simulink model "inverse_pendulum"  (R2016a)
settings: Solver=FixedStepAuto  StartTime=0.0  StopTime=inf  FixedStep=1e-4  RelTol=1e-3
undefined symbols (not defined in the file or in its folder): sigbuilder_block
libraries: fuzblock x6, simulink x2
settings Model: Creator=Salar Basiri  LastModifiedBy=Salar Basiri

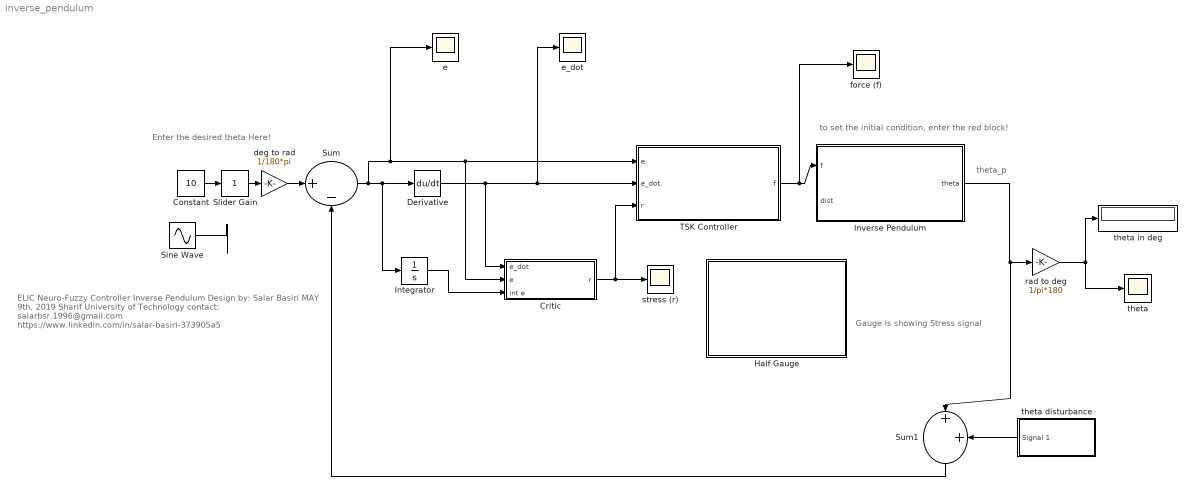
== system inverse_pendulum ==
  note: ELIC Neuro-Fuzzy Controller
      | Inverse Pendulum
      | Design by: Salar Basiri
      | MAY 9th, 2019
      | Sharif University of Technology
      | contact:
      | salarbsr.1996@gmail.com
      | https://www.linkedin.com/in/salar-basiri-373905a5
  note: to set the initial condition, enter the red block!
  note: Gauge is showing Stress signal
  note: Enter the desired theta Here!
  note: theta_p
  Constant : Constant  Value=10
  Critic : Subsystem
  Derivative : Derivative
  Half Gauge : Subsystem  DialogController=hmiCreateDDGDialog  IsWebBlock=on  mask(MWDashboardBlock){webBlockId=e21a16ba-fe41-4bad-9400-f35b9216ae1c, webBlockType=semicirculargauge, ShowInLibBrowser=on, ShowInitialText=on, HMISrcModelName=inverse_pendulum}
      mask prompts: webBlockId "WebBlock Id"; webBlockType "WebBlock Type"; HMISrcModelName "Source Model"
      mask Help: helpview([docroot '/mapfiles/simulink.map'], 'hmi_half_gauge')
      mask Display:
      | if strcmp(get_param(bdroot(gcb),'BlockDiagramType'), 'library')
      |     image([(matlabroot) '/toolbox/simulink/hmi/icons/SemicircularGauge.png']);
      | end
  Integrator : Integrator
  Inverse Pendulum : Subsystem
  Sine Wave : Sin  Amplitude=10  Frequency=5  SampleTime=0
  Slider Gain : simulink/Math Operations/Slider Gain  low=-1  gain=1  high=1
  Sum : Sum  Inputs=|+-
  Sum1 : Sum  Inputs=|++
  TSK Controller : Subsystem
  deg to rad : Gain  Gain=1/180*pi
  e : Scope
  e_dot : Scope
  force (f) : Scope
  rad to deg : Gain  Gain=1/pi*180
  stress (r) : Scope
  theta : Scope
  theta disturbance : Subsystem  Tag=STV Subsys  LoadFcn=sigbuilder_block('load');  StartFcn=sigbuilder_block('start');  StopFcn=sigbuilder_block('stop');  ClipboardFcn=sigbuilder_block('clipboard');  mask(Sigbuilder block){}
      mask help: Simulink:masks:SigbuilderBlock_MD
      mask init:
      | if ~strcmp(get_param(bdroot(gcbh),'SimulationStatus'),'stopped') tuvar = sigbuilder_block('maskInit'); end
      settings: CopyFcn=sigbuilder_block('copy');  DeleteFcn=sigbuilder_block('delete');  ModelCloseFcn=sigbuilder_block('modelClose');  PreSaveFcn=sigbuilder_block('preSave');  PauseFcn=sigbuilder_block('pause');  ContinueFcn=sigbuilder_block('continue');  NameChangeFcn=sigbuilder_block('namechange');  OpenFcn=sigbuilder_block('open',[6 30 1012.5 447.75 ]);  CloseFcn=sigbuilder_block('close');
      mask Display: plot(0, 0, 100, 100,[2, 2, 32, 32, 2], [68, 8, 8, 68, 68],[32, 2], [38, 38], [32, 19, 2],[53, 60, 44], [32, 17, 17, 2],[16, 16, 31, 31]);txt = getActiveGroup(gcbh);text(2, 100, txt,'verticalAlignment', 'top');
  theta in deg : Display
  wires:
  Inverse Pendulum/1(theta) -> Sum1/1, rad to deg/1
  Sum/1 -> Integrator/1, Derivative/1, e/1, Critic/2(e), TSK Controller/1(e)
  Derivative/1 -> Critic/1(e_dot), e_dot/1, TSK Controller/2(e_dot)
  TSK Controller/1(f) -> force (f)/1, Inverse Pendulum/1(f)
  rad to deg/1 -> theta/1, theta in deg/1
  deg to rad/1 -> Sum/1
  theta disturbance/1(Signal 1) -> Sum1/2
  Sum1/1 -> Sum/2
  Critic/1(r) -> TSK Controller/3(r), stress (r)/1
  Integrator/1 -> Critic/3(int e)
  Sine Wave/1 -> ?
  Slider Gain/1 -> deg to rad/1
  Constant/1 -> Slider Gain/1

== system inverse_pendulum/Critic ==
  e_dot : Inport
  e : Inport  Port=2
  int e : Inport  Port=3
  Constant : Constant  Value=20
  Constant1 : Constant  Value=5
  Constant2 : Constant  Value=10
  Product : Product
  Product1 : Product
  Product2 : Product
  Sum : Sum  Inputs=|+++
  r : Outport
  wires:
  Constant/1 -> Product/1
  e/1 -> Product/2
  e_dot/1 -> Product1/1
  Constant1/1 -> Product1/2
  Product/1 -> Sum/1
  Product1/1 -> Sum/2
  Sum/1 -> r/1
  int e/1 -> Product2/2
  Constant2/1 -> Product2/1
  Product2/1 -> Sum/3

== system inverse_pendulum/Half Gauge ==

== system inverse_pendulum/Inverse Pendulum ==
  note: set the initial conditions HERE!
  f : Inport
  dist : Inport  Port=2
  "Integrator, Second-Order" : SecondOrderIntegrator  ICX=0  ICDXDT=10/180*pi
  MATLAB Function : MATLAB Function  TreatAsAtomicUnit=on
  theta : Outport
  wires:
  "Integrator, Second-Order"/1 -> MATLAB Function/1(theta), theta/1
  "Integrator, Second-Order"/2 -> MATLAB Function/2(theta_p)
  f/1 -> MATLAB Function/3(f)
  MATLAB Function/1(theta_pp) -> "Integrator, Second-Order"/1
  dist/1 -> MATLAB Function/4(dist)

== system inverse_pendulum/TSK Controller ==
  e : Inport
  e_dot : Inport  Port=2
  r : Inport  Port=3
  Bus Creator : BusCreator  Inputs=3
  Subsystem : Subsystem
  Subsystem1 : Subsystem
  Subsystem10 : Subsystem
  Subsystem2 : Subsystem
  Subsystem3 : Subsystem
  Subsystem4 : Subsystem
  Subsystem5 : Subsystem
  Subsystem6 : Subsystem
  Subsystem7 : Subsystem
  Subsystem8 : Subsystem
  Subsystem9 : Subsystem
  Sum : Sum  Inputs=|+++++++++
  force limit : Saturate  UpperLimit=5  LowerLimit=-5
  f : Outport
  wires:
  e/1 -> Subsystem2/3(e), Subsystem8/3(e), Subsystem9/3(e), Subsystem10/3(e), Subsystem7/3(e), Subsystem6/3(e), Subsystem5/3(e), Subsystem4/3(e), Subsystem3/3(e), Subsystem1/2(e), Subsystem/1(e)
  e_dot/1 -> Subsystem3/4(e_dot), Subsystem5/4(e_dot), Subsystem6/4(e_dot), Subsystem7/4(e_dot), Subsystem8/4(e_dot), Subsystem10/4(e_dot), Subsystem9/4(e_dot), Subsystem4/4(e_dot), Subsystem2/4(e_dot), Subsystem/2(e_dot), Subsystem1/3(e_dot)
  r/1 -> Subsystem1/1(r)
  Subsystem/1(rule1) -> Subsystem2/1(myu)
  Subsystem1/1(a) -> Bus Creator/1
  Subsystem1/2(b) -> Bus Creator/2
  Subsystem1/3(c) -> Bus Creator/3
  Bus Creator/1 -> Subsystem5/2("mux "), Subsystem6/2("mux "), Subsystem8/2("mux "), Subsystem10/2("mux "), Subsystem9/2("mux "), Subsystem7/2("mux "), Subsystem3/2("mux "), Subsystem4/2("mux "), Subsystem2/2("mux ")
  Subsystem/2(rule2) -> Subsystem3/1(myu)
  Subsystem/3(rule3) -> Subsystem4/1(myu)
  Subsystem/4(rule4) -> Subsystem5/1(myu)
  Subsystem/5(rule5) -> Subsystem6/1(myu)
  Subsystem/6(rule6) -> Subsystem7/1(myu)
  Subsystem/7(rule7) -> Subsystem8/1(myu)
  Subsystem/8(rule8) -> Subsystem9/1(myu)
  Subsystem/9(rule9) -> Subsystem10/1(myu)
  Subsystem3/1(f) -> Sum/1
  Subsystem4/1(f) -> Sum/2
  Subsystem5/1(f) -> Sum/3
  Subsystem6/1(f) -> Sum/4
  Subsystem7/1(f) -> Sum/5
  Subsystem8/1(f) -> Sum/6
  Subsystem2/1(f) -> Sum/7
  Subsystem9/1(f) -> Sum/8
  Subsystem10/1(f) -> Sum/9
  Sum/1 -> force limit/1
  force limit/1 -> f/1

== system inverse_pendulum/theta disturbance ==
  Demux : Demux  Tag=STV Demux  Outputs=1
  FromWs : FromWorkspace  Tag=STV FromWs  VariableName=tuvar  SampleTime=0
      SigBuilderData=|
      | common.afterFinalStr = 'Extrapolate'
      | common.sampleTime = 0
      | dataSet.timeRange = [0 10]
      | dataSet.name = 'Group 1'
      | sbobj.Groups.Name = 'Group 1'
      | sbobj.Groups.Signals.Name = 'Signal 1'
      | sbobj.Groups.Signals.XData = [0 2 5 10]
      | sbobj.Groups.Signals.YData = [0 0 0 0]
  Signal 1 : Outport  Tag=STV Outport
  wires:
  Demux/1 -> Signal 1/1
  FromWs/1 -> Demux/1

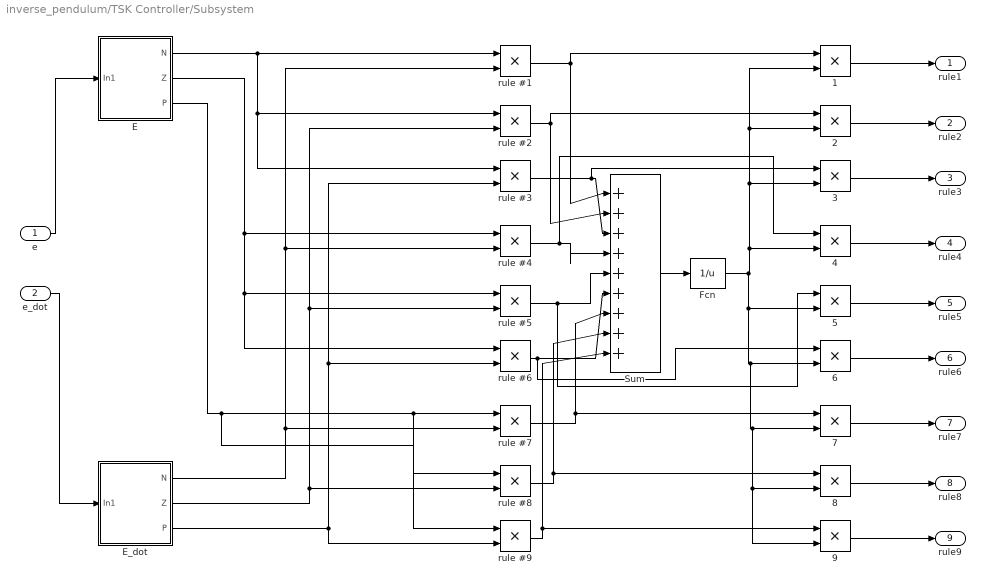
== system inverse_pendulum/TSK Controller/Subsystem ==
  e : Inport
  e_dot : Inport  Port=2
  {1..9} (9 alike) : Product
  E : Subsystem
  E_dot : Subsystem
  Fcn : Fcn  Expr=1/u
  Sum : Sum  Inputs=|+++++++++
  rule #{1..9} (9 alike) : Product
  rule1 : Outport
  rule2 : Outport  Port=2
  rule3 : Outport  Port=3
  rule4 : Outport  Port=4
  rule5 : Outport  Port=5
  rule6 : Outport  Port=6
  rule7 : Outport  Port=7
  rule8 : Outport  Port=8
  rule9 : Outport  Port=9
  wires:
  E_dot/1(N) -> rule #7/2, rule #4/2, rule #1/2
  E_dot/3(P) -> rule #6/2, rule #3/2, rule #9/2
  E/2(Z) -> rule #4/1, rule #5/1, rule #6/1
  E/1(N) -> rule #3/1, rule #2/1, rule #1/1
  E_dot/2(Z) -> rule #8/2, rule #5/2, rule #2/2
  E/3(P) -> rule #9/1, rule #8/1, rule #7/1
  e/1 -> E/1(In1)
  e_dot/1 -> E_dot/1(In1)
  rule #1/1 -> Sum/1, 1/1
  rule #2/1 -> Sum/2, 2/1
  rule #3/1 -> 3/1, Sum/3
  rule #4/1 -> 4/1, Sum/4
  rule #5/1 -> 5/1, Sum/5
  rule #6/1 -> 6/1, Sum/6
  rule #7/1 -> 7/1, Sum/7
  rule #8/1 -> 8/1, Sum/8
  rule #9/1 -> 9/1, Sum/9
  Sum/1 -> Fcn/1
  1/1 -> rule1/1
  2/1 -> rule2/1
  3/1 -> rule3/1
  4/1 -> rule4/1
  5/1 -> rule5/1
  6/1 -> rule6/1
  7/1 -> rule7/1
  8/1 -> rule8/1
  9/1 -> rule9/1
  Fcn/1 -> 9/2, 8/2, 7/2, 6/2, 5/2, 4/2, 3/2, 2/2, 1/2

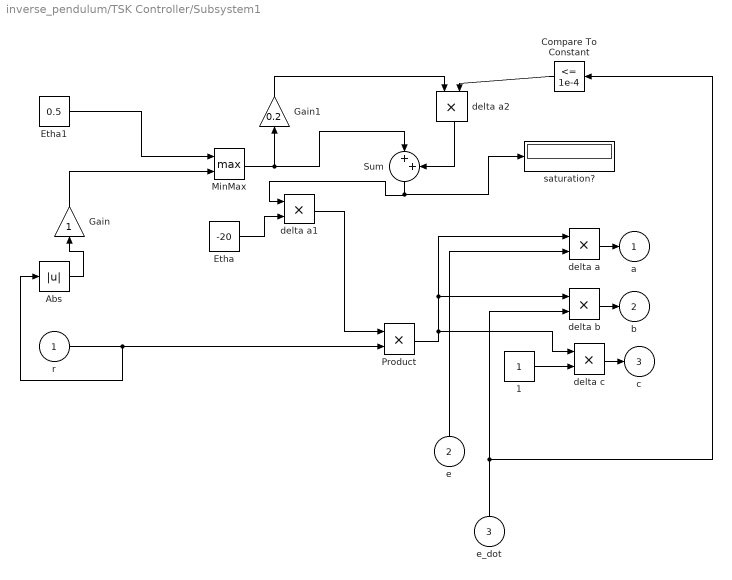
== system inverse_pendulum/TSK Controller/Subsystem1 ==
  r : Inport
  e : Inport  Port=2
  e_dot : Inport  Port=3
  1 : Constant
  Abs : Abs
  Compare To Constant : simulink/Logic and Bit Operations/Compare To Constant  relop=<=  const=1e-4  OutDataTypeStr=boolean
  Etha : Constant  Value=-20
  Etha1 : Constant  Value=0.5
  Gain : Gain
  Gain1 : Gain  Gain=0.2
  MinMax : MinMax  Function=max  Inputs=2
  Product : Product
  Sum : Sum  Inputs=|++
  delta a : Product
  delta a1 : Product
  delta a2 : Product
  "delta b " : Product
  delta c : Product
  saturation? : Display
  a : Outport
  b : Outport  Port=2
  c : Outport  Port=3
  wires:
  e_dot/1 -> Compare To Constant/1, "delta b "/2
  "delta b "/1 -> b/1
  e/1 -> delta a/2
  delta c/1 -> c/1
  delta a/1 -> a/1
  Product/1 -> delta a/1, "delta b "/1, delta c/1
  1/1 -> delta c/2
  r/1 -> Product/2, Abs/1
  Etha1/1 -> MinMax/1
  Etha/1 -> delta a1/2
  delta a1/1 -> Product/1
  Abs/1 -> Gain/1
  Gain/1 -> MinMax/2
  Compare To Constant/1 -> delta a2/2
  MinMax/1 -> Sum/1, Gain1/1
  Gain1/1 -> delta a2/1
  delta a2/1 -> Sum/2
  Sum/1 -> saturation?/1, delta a1/1

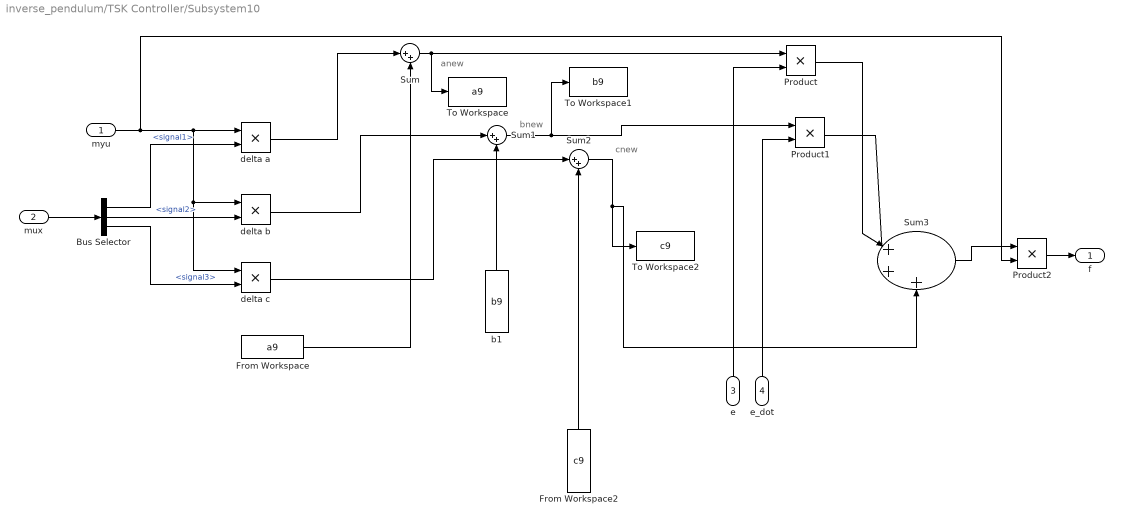
== system inverse_pendulum/TSK Controller/Subsystem10 ==
  note: cnew
  note: bnew
  note: anew
  myu : Inport
  "mux " : Inport  Port=2
  e : Inport  Port=3
  e_dot : Inport  Port=4
  Bus Selector : BusSelector
  From Workspace : FromWorkspace  VariableName=a9  SampleTime=0
  From Workspace2 : FromWorkspace  VariableName=c9  SampleTime=0
  Product : Product
  Product1 : Product
  Product2 : Product
  Sum : Sum  Inputs=|++
  Sum1 : Sum  Inputs=|++
  Sum2 : Sum  Inputs=|++
  Sum3 : Sum  Inputs=|+++
  To Workspace : ToWorkspace  VariableName=a9  SaveFormat=Timeseries  SampleTime=-1
  To Workspace1 : ToWorkspace  VariableName=b9  SaveFormat=Timeseries  SampleTime=-1
  To Workspace2 : ToWorkspace  VariableName=c9  SaveFormat=Timeseries  SampleTime=-1
  b1 : FromWorkspace  VariableName=b9  SampleTime=0
  delta a : Product
  delta b : Product
  delta c : Product
  f : Outport
  wires:
  myu/1 -> delta c/1, delta b/1, delta a/1, Product2/2
  delta a/1 -> Sum/1
  delta b/1 -> Sum1/1
  delta c/1 -> Sum2/1
  Sum1/1 -> To Workspace1/1, Product1/1
  Sum2/1 -> To Workspace2/1, Sum3/3
  "mux "/1 -> Bus Selector/1
  Bus Selector/1 -> delta a/2  "<signal1>"
  Bus Selector/2 -> delta b/2  "<signal2>"
  Bus Selector/3 -> delta c/2  "<signal3>"
  e/1 -> Product/2
  e_dot/1 -> Product1/2
  Product/1 -> Sum3/1
  Product1/1 -> Sum3/2
  Product2/1 -> f/1
  Sum3/1 -> Product2/1
  Sum/1 -> Product/1, To Workspace/1
  From Workspace/1 -> Sum/2
  b1/1 -> Sum1/2
  From Workspace2/1 -> Sum2/2

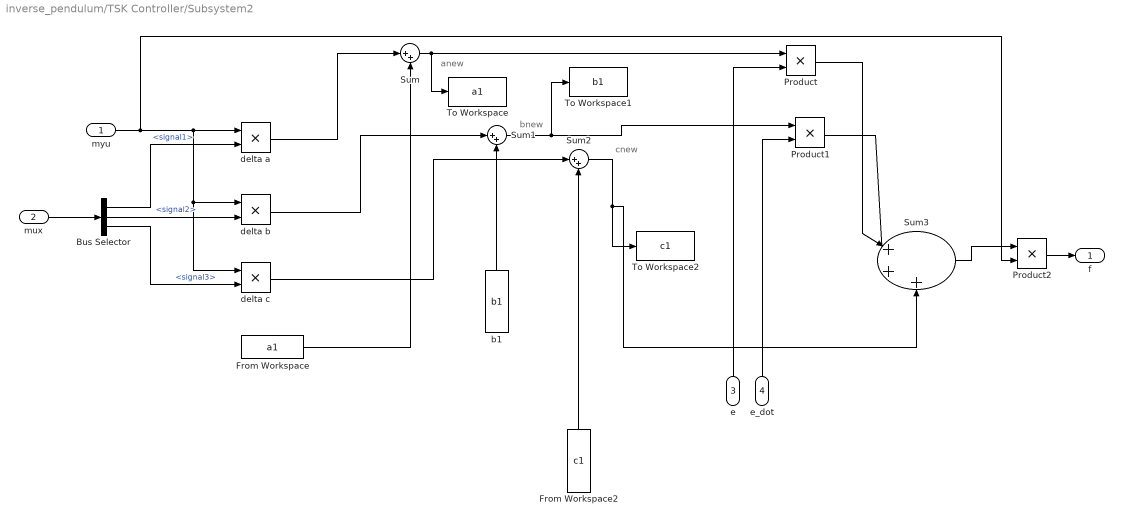
== system inverse_pendulum/TSK Controller/Subsystem2 ==
  note: cnew
  note: bnew
  note: anew
  myu : Inport
  "mux " : Inport  Port=2
  e : Inport  Port=3
  e_dot : Inport  Port=4
  Bus Selector : BusSelector
  From Workspace : FromWorkspace  VariableName=a1  SampleTime=0
  From Workspace2 : FromWorkspace  VariableName=c1  SampleTime=0
  Product : Product
  Product1 : Product
  Product2 : Product
  Sum : Sum  Inputs=|++
  Sum1 : Sum  Inputs=|++
  Sum2 : Sum  Inputs=|++
  Sum3 : Sum  Inputs=|+++
  To Workspace : ToWorkspace  VariableName=a1  SaveFormat=Timeseries  SampleTime=-1
  To Workspace1 : ToWorkspace  VariableName=b1  SaveFormat=Timeseries  SampleTime=-1
  To Workspace2 : ToWorkspace  VariableName=c1  SaveFormat=Timeseries  SampleTime=-1
  b1 : FromWorkspace  VariableName=b1  SampleTime=0
  delta a : Product
  delta b : Product
  delta c : Product
  f : Outport
  wires:
  myu/1 -> delta c/1, delta b/1, delta a/1, Product2/2
  delta a/1 -> Sum/1
  delta b/1 -> Sum1/1
  delta c/1 -> Sum2/1
  Sum1/1 -> To Workspace1/1, Product1/1
  Sum2/1 -> To Workspace2/1, Sum3/3
  "mux "/1 -> Bus Selector/1
  Bus Selector/1 -> delta a/2  "<signal1>"
  Bus Selector/2 -> delta b/2  "<signal2>"
  Bus Selector/3 -> delta c/2  "<signal3>"
  e/1 -> Product/2
  e_dot/1 -> Product1/2
  Product/1 -> Sum3/1
  Product1/1 -> Sum3/2
  Product2/1 -> f/1
  Sum3/1 -> Product2/1
  Sum/1 -> Product/1, To Workspace/1
  From Workspace/1 -> Sum/2
  b1/1 -> Sum1/2
  From Workspace2/1 -> Sum2/2

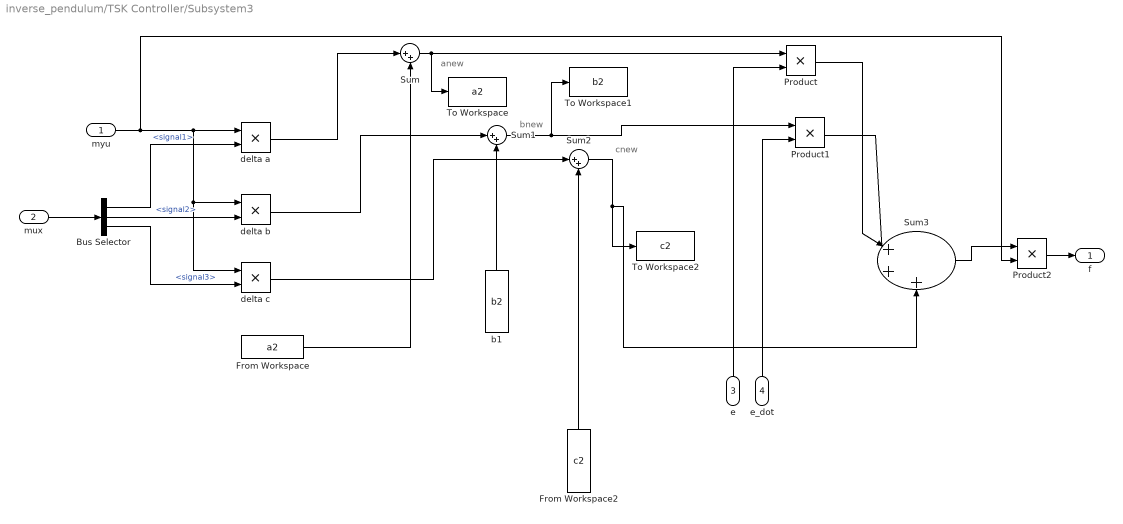
== system inverse_pendulum/TSK Controller/Subsystem3 ==
  note: cnew
  note: bnew
  note: anew
  myu : Inport
  "mux " : Inport  Port=2
  e : Inport  Port=3
  e_dot : Inport  Port=4
  Bus Selector : BusSelector
  From Workspace : FromWorkspace  VariableName=a2  SampleTime=0
  From Workspace2 : FromWorkspace  VariableName=c2  SampleTime=0
  Product : Product
  Product1 : Product
  Product2 : Product
  Sum : Sum  Inputs=|++
  Sum1 : Sum  Inputs=|++
  Sum2 : Sum  Inputs=|++
  Sum3 : Sum  Inputs=|+++
  To Workspace : ToWorkspace  VariableName=a2  SaveFormat=Timeseries  SampleTime=-1
  To Workspace1 : ToWorkspace  VariableName=b2  SaveFormat=Timeseries  SampleTime=-1
  To Workspace2 : ToWorkspace  VariableName=c2  SaveFormat=Timeseries  SampleTime=-1
  b1 : FromWorkspace  VariableName=b2  SampleTime=0
  delta a : Product
  delta b : Product
  delta c : Product
  f : Outport
  wires:
  myu/1 -> delta c/1, delta b/1, delta a/1, Product2/2
  delta a/1 -> Sum/1
  delta b/1 -> Sum1/1
  delta c/1 -> Sum2/1
  Sum1/1 -> To Workspace1/1, Product1/1
  Sum2/1 -> To Workspace2/1, Sum3/3
  "mux "/1 -> Bus Selector/1
  Bus Selector/1 -> delta a/2  "<signal1>"
  Bus Selector/2 -> delta b/2  "<signal2>"
  Bus Selector/3 -> delta c/2  "<signal3>"
  e/1 -> Product/2
  e_dot/1 -> Product1/2
  Product/1 -> Sum3/1
  Product1/1 -> Sum3/2
  Product2/1 -> f/1
  Sum3/1 -> Product2/1
  Sum/1 -> Product/1, To Workspace/1
  From Workspace/1 -> Sum/2
  b1/1 -> Sum1/2
  From Workspace2/1 -> Sum2/2

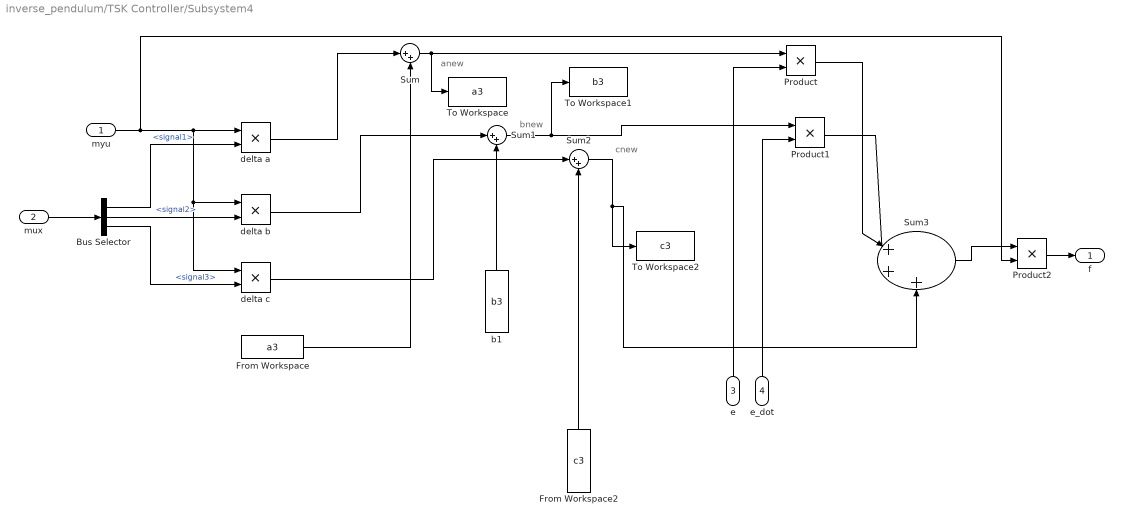
== system inverse_pendulum/TSK Controller/Subsystem4 ==
  note: cnew
  note: bnew
  note: anew
  myu : Inport
  "mux " : Inport  Port=2
  e : Inport  Port=3
  e_dot : Inport  Port=4
  Bus Selector : BusSelector
  From Workspace : FromWorkspace  VariableName=a3  SampleTime=0
  From Workspace2 : FromWorkspace  VariableName=c3  SampleTime=0
  Product : Product
  Product1 : Product
  Product2 : Product
  Sum : Sum  Inputs=|++
  Sum1 : Sum  Inputs=|++
  Sum2 : Sum  Inputs=|++
  Sum3 : Sum  Inputs=|+++
  To Workspace : ToWorkspace  VariableName=a3  SaveFormat=Timeseries  SampleTime=-1
  To Workspace1 : ToWorkspace  VariableName=b3  SaveFormat=Timeseries  SampleTime=-1
  To Workspace2 : ToWorkspace  VariableName=c3  SaveFormat=Timeseries  SampleTime=-1
  b1 : FromWorkspace  VariableName=b3  SampleTime=0
  delta a : Product
  delta b : Product
  delta c : Product
  f : Outport
  wires:
  myu/1 -> delta c/1, delta b/1, delta a/1, Product2/2
  delta a/1 -> Sum/1
  delta b/1 -> Sum1/1
  delta c/1 -> Sum2/1
  Sum1/1 -> To Workspace1/1, Product1/1
  Sum2/1 -> To Workspace2/1, Sum3/3
  "mux "/1 -> Bus Selector/1
  Bus Selector/1 -> delta a/2  "<signal1>"
  Bus Selector/2 -> delta b/2  "<signal2>"
  Bus Selector/3 -> delta c/2  "<signal3>"
  e/1 -> Product/2
  e_dot/1 -> Product1/2
  Product/1 -> Sum3/1
  Product1/1 -> Sum3/2
  Product2/1 -> f/1
  Sum3/1 -> Product2/1
  Sum/1 -> Product/1, To Workspace/1
  From Workspace/1 -> Sum/2
  b1/1 -> Sum1/2
  From Workspace2/1 -> Sum2/2

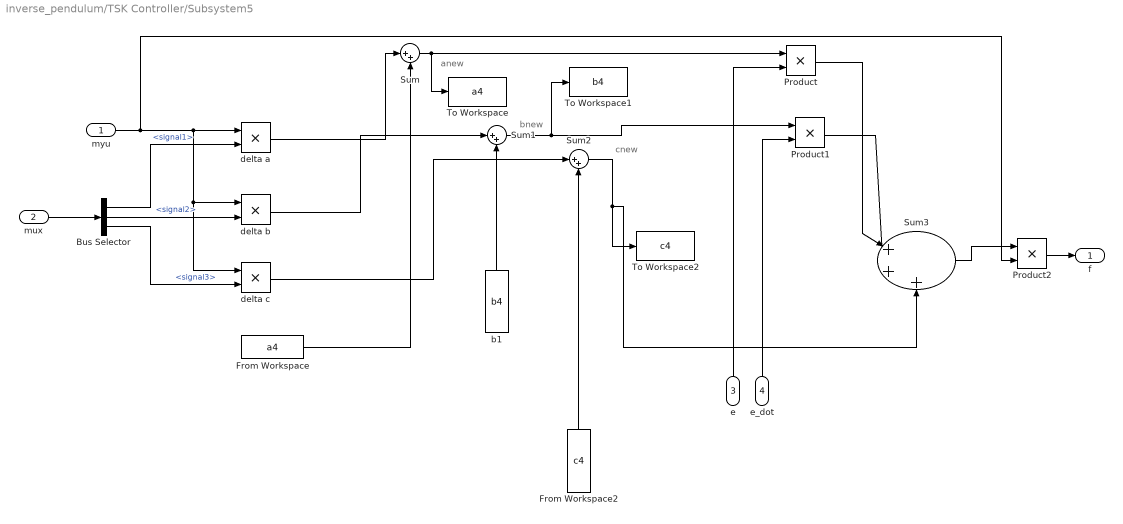
== system inverse_pendulum/TSK Controller/Subsystem5 ==
  note: cnew
  note: bnew
  note: anew
  myu : Inport
  "mux " : Inport  Port=2
  e : Inport  Port=3
  e_dot : Inport  Port=4
  Bus Selector : BusSelector
  From Workspace : FromWorkspace  VariableName=a4  SampleTime=0
  From Workspace2 : FromWorkspace  VariableName=c4  SampleTime=0
  Product : Product
  Product1 : Product
  Product2 : Product
  Sum : Sum  Inputs=|++
  Sum1 : Sum  Inputs=|++
  Sum2 : Sum  Inputs=|++
  Sum3 : Sum  Inputs=|+++
  To Workspace : ToWorkspace  VariableName=a4  SaveFormat=Timeseries  SampleTime=-1
  To Workspace1 : ToWorkspace  VariableName=b4  SaveFormat=Timeseries  SampleTime=-1
  To Workspace2 : ToWorkspace  VariableName=c4  SaveFormat=Timeseries  SampleTime=-1
  b1 : FromWorkspace  VariableName=b4  SampleTime=0
  delta a : Product
  delta b : Product
  delta c : Product
  f : Outport
  wires:
  myu/1 -> delta c/1, delta b/1, delta a/1, Product2/2
  delta a/1 -> Sum/1
  delta b/1 -> Sum1/1
  delta c/1 -> Sum2/1
  Sum1/1 -> To Workspace1/1, Product1/1
  Sum2/1 -> To Workspace2/1, Sum3/3
  "mux "/1 -> Bus Selector/1
  Bus Selector/1 -> delta a/2  "<signal1>"
  Bus Selector/2 -> delta b/2  "<signal2>"
  Bus Selector/3 -> delta c/2  "<signal3>"
  e/1 -> Product/2
  e_dot/1 -> Product1/2
  Product/1 -> Sum3/1
  Product1/1 -> Sum3/2
  Product2/1 -> f/1
  Sum3/1 -> Product2/1
  Sum/1 -> Product/1, To Workspace/1
  From Workspace/1 -> Sum/2
  b1/1 -> Sum1/2
  From Workspace2/1 -> Sum2/2

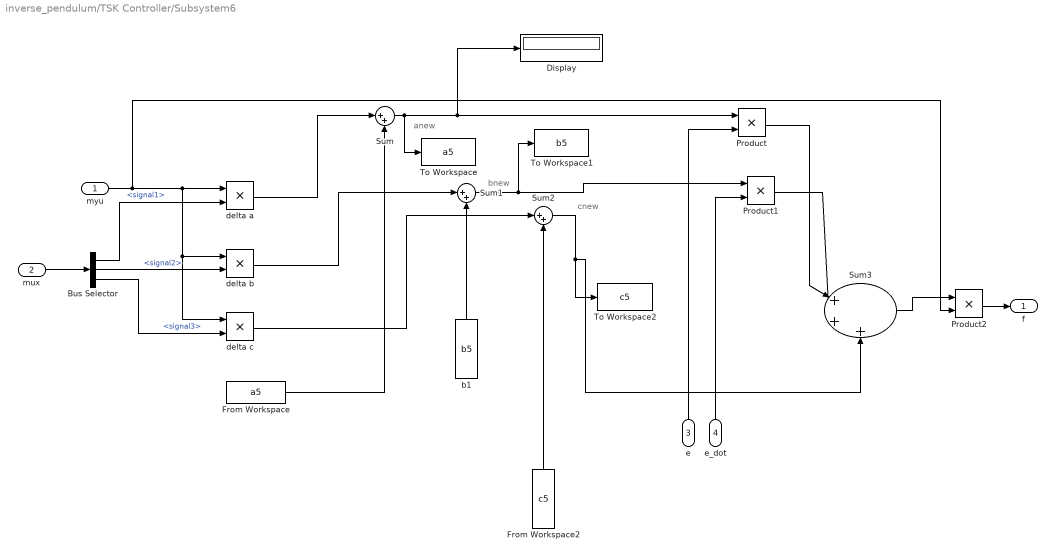
== system inverse_pendulum/TSK Controller/Subsystem6 ==
  note: cnew
  note: bnew
  note: anew
  myu : Inport
  "mux " : Inport  Port=2
  e : Inport  Port=3
  e_dot : Inport  Port=4
  Bus Selector : BusSelector
  Display : Display
  From Workspace : FromWorkspace  VariableName=a5  SampleTime=0
  From Workspace2 : FromWorkspace  VariableName=c5  SampleTime=0
  Product : Product
  Product1 : Product
  Product2 : Product
  Sum : Sum  Inputs=|++
  Sum1 : Sum  Inputs=|++
  Sum2 : Sum  Inputs=|++
  Sum3 : Sum  Inputs=|+++
  To Workspace : ToWorkspace  VariableName=a5  SaveFormat=Timeseries  SampleTime=-1
  To Workspace1 : ToWorkspace  VariableName=b5  SaveFormat=Timeseries  SampleTime=-1
  To Workspace2 : ToWorkspace  VariableName=c5  SaveFormat=Timeseries  SampleTime=-1
  b1 : FromWorkspace  VariableName=b5  SampleTime=0
  delta a : Product
  delta b : Product
  delta c : Product
  f : Outport
  wires:
  myu/1 -> delta c/1, delta b/1, delta a/1, Product2/2
  delta a/1 -> Sum/1
  delta b/1 -> Sum1/1
  delta c/1 -> Sum2/1
  Sum1/1 -> To Workspace1/1, Product1/1
  Sum2/1 -> To Workspace2/1, Sum3/3
  "mux "/1 -> Bus Selector/1
  Bus Selector/1 -> delta a/2  "<signal1>"
  Bus Selector/2 -> delta b/2  "<signal2>"
  Bus Selector/3 -> delta c/2  "<signal3>"
  e/1 -> Product/2
  e_dot/1 -> Product1/2
  Product/1 -> Sum3/1
  Product1/1 -> Sum3/2
  Product2/1 -> f/1
  Sum3/1 -> Product2/1
  Sum/1 -> Display/1, Product/1, To Workspace/1
  From Workspace/1 -> Sum/2
  b1/1 -> Sum1/2
  From Workspace2/1 -> Sum2/2

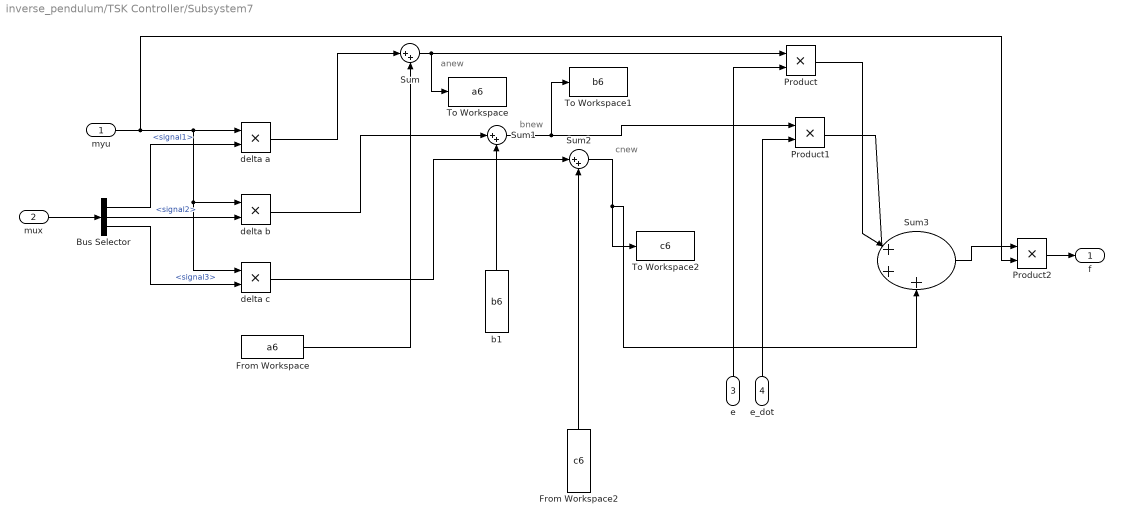
== system inverse_pendulum/TSK Controller/Subsystem7 ==
  note: cnew
  note: bnew
  note: anew
  myu : Inport
  "mux " : Inport  Port=2
  e : Inport  Port=3
  e_dot : Inport  Port=4
  Bus Selector : BusSelector
  From Workspace : FromWorkspace  VariableName=a6  SampleTime=0
  From Workspace2 : FromWorkspace  VariableName=c6  SampleTime=0
  Product : Product
  Product1 : Product
  Product2 : Product
  Sum : Sum  Inputs=|++
  Sum1 : Sum  Inputs=|++
  Sum2 : Sum  Inputs=|++
  Sum3 : Sum  Inputs=|+++
  To Workspace : ToWorkspace  VariableName=a6  SaveFormat=Timeseries  SampleTime=-1
  To Workspace1 : ToWorkspace  VariableName=b6  SaveFormat=Timeseries  SampleTime=-1
  To Workspace2 : ToWorkspace  VariableName=c6  SaveFormat=Timeseries  SampleTime=-1
  b1 : FromWorkspace  VariableName=b6  SampleTime=0
  delta a : Product
  delta b : Product
  delta c : Product
  f : Outport
  wires:
  myu/1 -> delta c/1, delta b/1, delta a/1, Product2/2
  delta a/1 -> Sum/1
  delta b/1 -> Sum1/1
  delta c/1 -> Sum2/1
  Sum1/1 -> To Workspace1/1, Product1/1
  Sum2/1 -> To Workspace2/1, Sum3/3
  "mux "/1 -> Bus Selector/1
  Bus Selector/1 -> delta a/2  "<signal1>"
  Bus Selector/2 -> delta b/2  "<signal2>"
  Bus Selector/3 -> delta c/2  "<signal3>"
  e/1 -> Product/2
  e_dot/1 -> Product1/2
  Product/1 -> Sum3/1
  Product1/1 -> Sum3/2
  Product2/1 -> f/1
  Sum3/1 -> Product2/1
  Sum/1 -> Product/1, To Workspace/1
  From Workspace/1 -> Sum/2
  b1/1 -> Sum1/2
  From Workspace2/1 -> Sum2/2

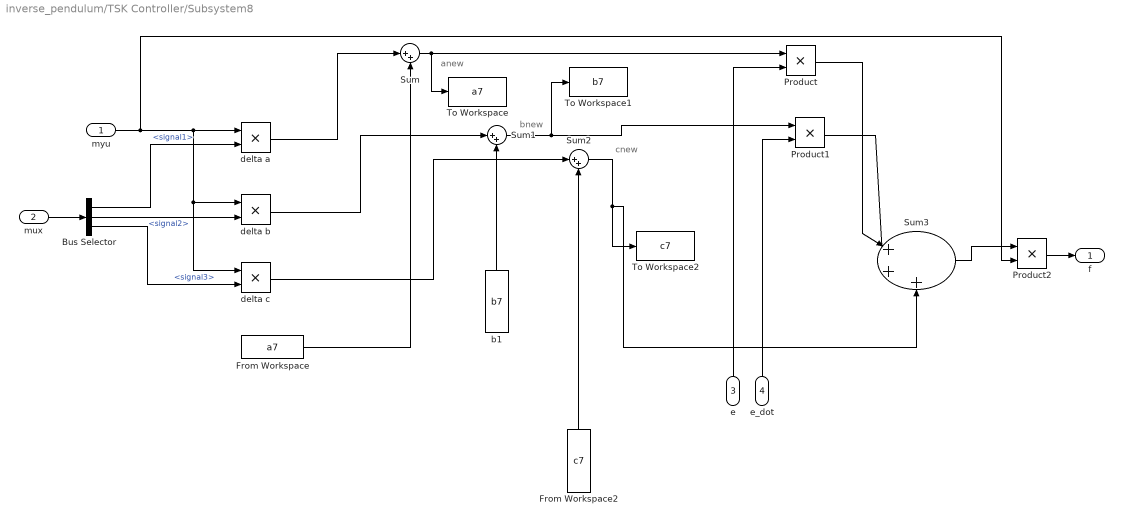
== system inverse_pendulum/TSK Controller/Subsystem8 ==
  note: cnew
  note: bnew
  note: anew
  myu : Inport
  "mux " : Inport  Port=2
  e : Inport  Port=3
  e_dot : Inport  Port=4
  Bus Selector : BusSelector
  From Workspace : FromWorkspace  VariableName=a7  SampleTime=0
  From Workspace2 : FromWorkspace  VariableName=c7  SampleTime=0
  Product : Product
  Product1 : Product
  Product2 : Product
  Sum : Sum  Inputs=|++
  Sum1 : Sum  Inputs=|++
  Sum2 : Sum  Inputs=|++
  Sum3 : Sum  Inputs=|+++
  To Workspace : ToWorkspace  VariableName=a7  SaveFormat=Timeseries  SampleTime=-1
  To Workspace1 : ToWorkspace  VariableName=b7  SaveFormat=Timeseries  SampleTime=-1
  To Workspace2 : ToWorkspace  VariableName=c7  SaveFormat=Timeseries  SampleTime=-1
  b1 : FromWorkspace  VariableName=b7  SampleTime=0
  delta a : Product
  delta b : Product
  delta c : Product
  f : Outport
  wires:
  myu/1 -> delta c/1, delta b/1, delta a/1, Product2/2
  delta a/1 -> Sum/1
  delta b/1 -> Sum1/1
  delta c/1 -> Sum2/1
  Sum1/1 -> To Workspace1/1, Product1/1
  Sum2/1 -> To Workspace2/1, Sum3/3
  "mux "/1 -> Bus Selector/1
  Bus Selector/1 -> delta a/2  "<signal1>"
  Bus Selector/2 -> delta b/2  "<signal2>"
  Bus Selector/3 -> delta c/2  "<signal3>"
  e/1 -> Product/2
  e_dot/1 -> Product1/2
  Product/1 -> Sum3/1
  Product1/1 -> Sum3/2
  Product2/1 -> f/1
  Sum3/1 -> Product2/1
  Sum/1 -> Product/1, To Workspace/1
  From Workspace/1 -> Sum/2
  b1/1 -> Sum1/2
  From Workspace2/1 -> Sum2/2

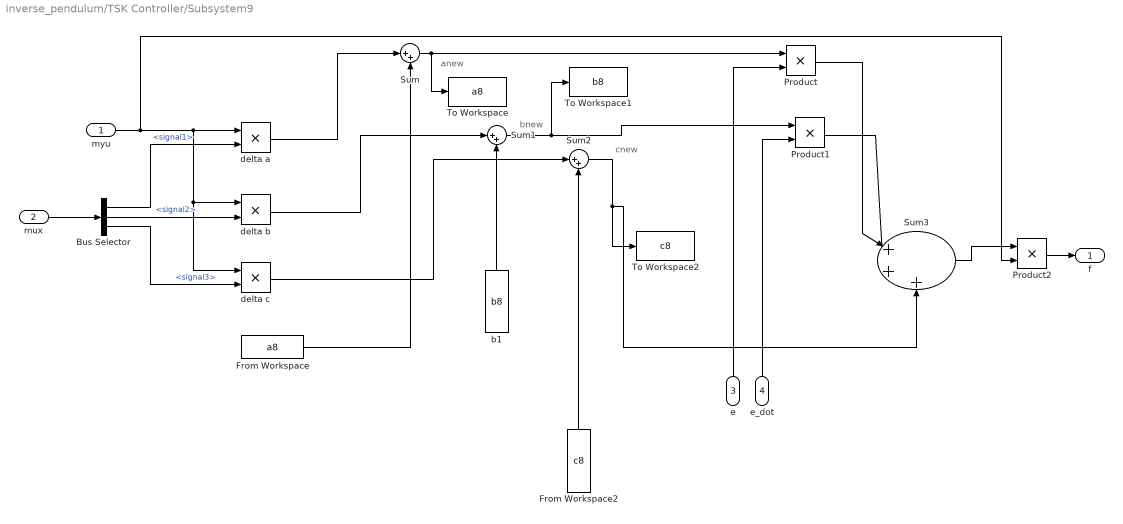
== system inverse_pendulum/TSK Controller/Subsystem9 ==
  note: cnew
  note: bnew
  note: anew
  myu : Inport
  "mux " : Inport  Port=2
  e : Inport  Port=3
  e_dot : Inport  Port=4
  Bus Selector : BusSelector
  From Workspace : FromWorkspace  VariableName=a8  SampleTime=0
  From Workspace2 : FromWorkspace  VariableName=c8  SampleTime=0
  Product : Product
  Product1 : Product
  Product2 : Product
  Sum : Sum  Inputs=|++
  Sum1 : Sum  Inputs=|++
  Sum2 : Sum  Inputs=|++
  Sum3 : Sum  Inputs=|+++
  To Workspace : ToWorkspace  VariableName=a8  SaveFormat=Timeseries  SampleTime=-1
  To Workspace1 : ToWorkspace  VariableName=b8  SaveFormat=Timeseries  SampleTime=-1
  To Workspace2 : ToWorkspace  VariableName=c8  SaveFormat=Timeseries  SampleTime=-1
  b1 : FromWorkspace  VariableName=b8  SampleTime=0
  delta a : Product
  delta b : Product
  delta c : Product
  f : Outport
  wires:
  myu/1 -> delta c/1, delta b/1, delta a/1, Product2/2
  delta a/1 -> Sum/1
  delta b/1 -> Sum1/1
  delta c/1 -> Sum2/1
  Sum1/1 -> To Workspace1/1, Product1/1
  Sum2/1 -> To Workspace2/1, Sum3/3
  "mux "/1 -> Bus Selector/1
  Bus Selector/1 -> delta a/2  "<signal1>"
  Bus Selector/2 -> delta b/2  "<signal2>"
  Bus Selector/3 -> delta c/2  "<signal3>"
  e/1 -> Product/2
  e_dot/1 -> Product1/2
  Product/1 -> Sum3/1
  Product1/1 -> Sum3/2
  Product2/1 -> f/1
  Sum3/1 -> Product2/1
  Sum/1 -> Product/1, To Workspace/1
  From Workspace/1 -> Sum/2
  b1/1 -> Sum1/2
  From Workspace2/1 -> Sum2/2

== system inverse_pendulum/TSK Controller/Subsystem/E ==
  In1 : Inport
  Display : Display
  Display1 : Display
  Display2 : Display
  NB : fuzblock/Membership  Functions/Trapezoidal MF  a=-inf  b=-inf  c=-10/180*pi  d=0
  PB : fuzblock/Membership  Functions/Trapezoidal MF  a=0  b=10/180*pi  c=inf  d=inf
  ZE : fuzblock/Membership  Functions/Triangular MF  a=-10/180*pi  b=0  c=10/180*pi
  N : Outport
  Z : Outport  Port=2
  P : Outport  Port=3
  wires:
  PB/1 -> Display2/1, P/1
  ZE/1 -> Display1/1, Z/1
  NB/1 -> Display/1, N/1
  In1/1 -> PB/1, ZE/1, NB/1

== system inverse_pendulum/TSK Controller/Subsystem/E_dot ==
  In1 : Inport
  Display : Display
  Display1 : Display
  Display2 : Display
  NB : fuzblock/Membership  Functions/Trapezoidal MF  a=-inf  b=-inf  c=-10/180*pi  d=0
  PB : fuzblock/Membership  Functions/Trapezoidal MF  a=0  b=10/180*pi  c=inf  d=inf
  ZE : fuzblock/Membership  Functions/Triangular MF  a=-10/180*pi  b=0  c=10/180*pi
  N : Outport
  Z : Outport  Port=2
  P : Outport  Port=3
  wires:
  PB/1 -> Display2/1, P/1
  ZE/1 -> Display1/1, Z/1
  NB/1 -> Display/1, N/1
  In1/1 -> PB/1, ZE/1, NB/1

== matlab function inverse_pendulum/Inverse Pendulum/MATLAB Function ==
  data: theta input; theta_pp output; theta_p input; f input; dist input
function theta_pp = fcn(theta,theta_p,f,dist)

mc=1;
m=0.1;
l=0.5;
g=9.81;


theta_pp=(g*sin(theta)+cos(theta)*(-(f+dist)-m*l*theta_p^2*sin(theta))/(mc+m))/(l*(4/3-m/(mc+m)*(cos(theta))^2));

end
